simulink library "LM_LIB"  (R2019b)
settings: Solver=VariableStepAuto  StartTime=0.0  StopTime=10.0  RelTol=1e-3
undefined symbols (not defined in the file): P_LM_FusBLParFiltP, P_LM_FusParC0Index, P_LM_FusParC1Index, P_LM_FusParC2Index, P_LM_FusParC3Index, P_LM_OTLBufTPMinPntNum, P_LM_OTLBufTPSPosMinDis, P_LM_OTLRearMaxDis, P_LM_OTLTPNum
libraries: simulink x84, $bdroot x3
(part 5 of 5)

== system LM_LIB/LM_OTLBufLostTPValidJudgeNew/If Action Subsystem/If Action Subsystem/If Action Subsystem ==
  LM_OTLBufSPPosK1 : Inport
  LM_OTLBufEPPosK1 : Inport  Port=2
  LM_OTLBufPNumK1 : Inport  Port=3
  Action Port : ActionPort  ActionPortLabel=if(u1 ~= 0)
  Constant1 : Constant  OutDataTypeStr=uint8
  LM_OTLBufLastTPValid : Outport
  LM_OTLBufLastPNum : Outport  Port=2
  LM_OTLBufLastSPPos : Outport  Port=3
  LM_OTLBufLastEPPos : Outport  Port=4
  wires:
  LM_OTLBufSPPosK1/1 -> LM_OTLBufLastSPPos/1  "LM_OTLBufLastSPPos"
  LM_OTLBufEPPosK1/1 -> LM_OTLBufLastEPPos/1  "LM_OTLBufLastEPPos"
  LM_OTLBufPNumK1/1 -> LM_OTLBufLastPNum/1  "LM_OTLBufLastPNum"
  Constant1/1 -> LM_OTLBufLastTPValid/1  "LM_OTLBufLastTPValid"

== system LM_LIB/LM_OTLBufLostTPValidJudgeNew/If Action Subsystem/If Action Subsystem/If Action Subsystem1 ==
  LM_OTLBufDxVectK1Adju : Inport
  LM_OTLBufLastPNumK1 : Inport  Port=2
  LM_OTLBufLastSPPosK1 : Inport  Port=3
  LM_OTLBufLastEPPosK1 : Inport  Port=4
  Action Port : ActionPort  ActionPortLabel=else
  LM_OTL_Last1ObjValidTPDisClac : Subsystem
  LM_OTL_Last2ObjTPValidJudge : Subsystem
  Subsystem2 : Subsystem
  LM_OTLBufLastTPValid : Outport
  LM_OTLBufLastPNum : Outport  Port=2
  LM_OTLBufLastSPPos : Outport  Port=3
  LM_OTLBufLastEPPos : Outport  Port=4
  wires:
  LM_OTLBufDxVectK1Adju/1 -> LM_OTL_Last1ObjValidTPDisClac/1(LM_OTLBufDxVectK1Adju)
  LM_OTLBufLastSPPosK1/1 -> Subsystem2/2(LM_OTLBufLastSPPosK1), LM_OTL_Last1ObjValidTPDisClac/2(LM_OTLBufLastSPPosK1)
  LM_OTLBufLastEPPosK1/1 -> Subsystem2/3(LM_OTLBufLastEPPosK1), LM_OTL_Last1ObjValidTPDisClac/3(LM_OTLBufLastEPPosK1)
  LM_OTL_Last1ObjValidTPDisClac/1(LM_OTLLast2ObjValidTPDis) -> LM_OTL_Last2ObjTPValidJudge/1(LM_OTLLast2ObjValidTPDis)
  LM_OTL_Last2ObjTPValidJudge/1(LM_OTLLast2ObjTPValid) -> Subsystem2/1(LM_OTLLast2ObjTPValid)
  LM_OTLBufLastPNumK1/1 -> Subsystem2/4(LM_OTLBufLastPNumK1)
  Subsystem2/1(LM_OTLBufLastTPValid) -> LM_OTLBufLastTPValid/1
  Subsystem2/2(LM_OTLBufLastPNum) -> LM_OTLBufLastPNum/1
  Subsystem2/3(LM_OTLBufLastSPPos) -> LM_OTLBufLastSPPos/1
  Subsystem2/4(LM_OTLBufLastEPPos) -> LM_OTLBufLastEPPos/1

== system LM_LIB/LM_OTLBufLostTPValidJudgeNew/If Action Subsystem/If Action Subsystem/LM_OTL_Last1ObjTPValidJudge ==
  LM_OTLLast1ObjValidTPDis : Inport
  Constant : Constant  Value=10  OutDataTypeStr=single
  Relational Operator : RelationalOperator  OutDataTypeStr=boolean  RndMeth=Simplest
  LM_OTLLast1ObjTPValid : Outport
  wires:
  Relational Operator/1 -> LM_OTLLast1ObjTPValid/1  "LM_OTLLast1ObjTPValid"
  Constant/1 -> Relational Operator/2
  LM_OTLLast1ObjValidTPDis/1 -> Relational Operator/1

== system LM_LIB/LM_OTLBufLostTPValidJudgeNew/If Action Subsystem/If Action Subsystem/LM_OTL_Last1ObjValidTPDisClac ==
  LM_OTLBufL1DxVectK1Adju : Inport
  LM_OTLBufSPPosK1 : Inport  Port=2
  LM_OTLBufEPPosK1 : Inport  Port=3
  Constant : Constant  Value=0  OutDataTypeStr=single
  Index Vector : MultiPortSwitch  Inputs=1
  Index Vector1 : MultiPortSwitch  Inputs=1
  Relational Operator : RelationalOperator  Operator=>  OutDataTypeStr=boolean  RndMeth=Simplest
  Saturation : Saturate  UpperLimit=80  LowerLimit=1
  Saturation1 : Saturate  UpperLimit=80  LowerLimit=1
  Subtract : Sum  Inputs=+-
  Switch : Switch  Criteria=u2 ~= 0
  LM_OTLLast1ObjValidTPDis : Outport
  wires:
  Relational Operator/1 -> Switch/2
  Switch/1 -> Subtract/2
  Index Vector1/1 -> Subtract/1  "EndDis"
  Index Vector/1 -> Switch/1, Relational Operator/1  "StartDis"
  LM_OTLBufEPPosK1/1 -> Saturation/1
  LM_OTLBufL1DxVectK1Adju/1 -> Index Vector1/2, Index Vector/2
  LM_OTLBufSPPosK1/1 -> Saturation1/1
  Subtract/1 -> LM_OTLLast1ObjValidTPDis/1  "LM_OTLLast1ObjValidTPDis"
  Constant/1 -> Relational Operator/2, Switch/3
  Saturation/1 -> Index Vector1/1
  Saturation1/1 -> Index Vector/1

== system LM_LIB/LM_OTLBufLostTPValidJudgeNew/If Action Subsystem/If Action Subsystem1/LM_OTL_Last1ObjTPValidJudge ==
  LM_OTLLast1ObjValidTPDis : Inport
  Constant : Constant  Value=10  OutDataTypeStr=single
  Relational Operator : RelationalOperator  OutDataTypeStr=boolean  RndMeth=Simplest
  LM_OTLLast1ObjTPValid : Outport
  wires:
  LM_OTLLast1ObjValidTPDis/1 -> Relational Operator/1
  Constant/1 -> Relational Operator/2
  Relational Operator/1 -> LM_OTLLast1ObjTPValid/1  "LM_OTLLast1ObjTPValid"

== system LM_LIB/LM_OTLBufLostTPValidJudgeNew/If Action Subsystem/If Action Subsystem1/LM_OTL_Last1ObjValidTPDisClac ==
  LM_OTLBufL1DxVectK1Adju : Inport
  LM_OTLBufSPPosK1 : Inport  Port=2
  LM_OTLBufEPPosK1 : Inport  Port=3
  Constant : Constant  Value=0  OutDataTypeStr=single
  Index Vector : MultiPortSwitch  Inputs=1
  Index Vector1 : MultiPortSwitch  Inputs=1
  Relational Operator : RelationalOperator  Operator=>  OutDataTypeStr=boolean  RndMeth=Simplest
  Saturation : Saturate  UpperLimit=80  LowerLimit=1
  Saturation1 : Saturate  UpperLimit=80  LowerLimit=1
  Subtract : Sum  Inputs=+-
  Switch : Switch  Criteria=u2 ~= 0
  LM_OTLLast1ObjValidTPDis : Outport
  wires:
  LM_OTLBufSPPosK1/1 -> Saturation1/1
  LM_OTLBufL1DxVectK1Adju/1 -> Index Vector1/2, Index Vector/2
  LM_OTLBufEPPosK1/1 -> Saturation/1
  Index Vector/1 -> Switch/1, Relational Operator/1  "StartDis"
  Constant/1 -> Relational Operator/2, Switch/3
  Relational Operator/1 -> Switch/2
  Index Vector1/1 -> Subtract/1  "EndDis"
  Switch/1 -> Subtract/2
  Subtract/1 -> LM_OTLLast1ObjValidTPDis/1  "LM_OTLLast1ObjValidTPDis"
  Saturation/1 -> Index Vector1/1
  Saturation1/1 -> Index Vector/1

== system LM_LIB/LM_OTLBufLostTPValidJudgeNew/If Action Subsystem/If Action Subsystem1/LM_OTL_LastObjInfoCalc ==
  LM_OTLLast1ObjTPValid : Inport
  LM_OTLBufSPPosK1 : Inport  Port=2
  LM_OTLBufEPPosK1 : Inport  Port=3
  LM_OTLBufPNumK1 : Inport  Port=4
  Constant1 : Constant  OutDataTypeStr=uint8
  Constant2 : Constant  Value=0  OutDataTypeStr=uint8
  Constant3 : Constant  Value=0  OutDataTypeStr=uint8
  Switch{,1..3} (4 alike) : Switch  Criteria=u2 ~= 0
  LM_OTLBufLastTPValid : Outport
  LM_OTLBufLastPNum : Outport  Port=2
  LM_OTLBufLastSPPos : Outport  Port=3
  LM_OTLBufLastEPPos : Outport  Port=4
  wires:
  LM_OTLLast1ObjTPValid/1 -> Switch3/2, Switch2/2, Switch/2, Switch1/2
  Constant2/1 -> Switch1/3
  Constant1/1 -> Switch1/1
  Switch1/1 -> LM_OTLBufLastTPValid/1  "LM_OTLBufLastTPValid"
  Switch/1 -> LM_OTLBufLastPNum/1  "LM_OTLBufLastPNum"
  LM_OTLBufPNumK1/1 -> Switch/1
  Constant3/1 -> Switch3/3, Switch2/3, Switch/3
  Switch2/1 -> LM_OTLBufLastSPPos/1  "LM_OTLBufLastSPPos"
  LM_OTLBufSPPosK1/1 -> Switch2/1
  Switch3/1 -> LM_OTLBufLastEPPos/1  "LM_OTLBufLastEPPos"
  LM_OTLBufEPPosK1/1 -> Switch3/1

== system LM_LIB/LM_OTL_Buf1InfoUpdate/LM_OTL_BufLe1StoreInfoCalc/LM_OTL_ObjSICCurLeObj1InBufLe1/LM_OTL_BufL1DxInfo ==
  LM_OTLCurLeLaObj1Dx : Inport
  LM_OTLCurLeLaObj1RcdFlg : Inport  Port=2
  Constant : Constant  Value=0  OutDataTypeStr=single
  Switch4 : Switch  Criteria=u2 ~= 0
  LM_OTLBufL1Objdx : Outport
  wires:
  LM_OTLCurLeLaObj1Dx/1 -> Switch4/1
  LM_OTLCurLeLaObj1RcdFlg/1 -> Switch4/2
  Switch4/1 -> LM_OTLBufL1Objdx/1  "LM_OTLBufL1Objdx"
  Constant/1 -> Switch4/3

== system LM_LIB/LM_OTL_Buf1InfoUpdate/LM_OTL_BufLe1StoreInfoCalc/LM_OTL_ObjSICCurLeObj1InBufLe1/LM_OTL_BufL1DyInfo ==
  LM_OTLCurLeLaObj1Dy : Inport
  LM_OTLCurLeLaObj1RcdFlg : Inport  Port=2
  Constant : Constant  Value=0  OutDataTypeStr=single
  Switch4 : Switch  Criteria=u2 ~= 0
  LM_OTLBufL1ObjDy : Outport
  wires:
  Constant/1 -> Switch4/3
  Switch4/1 -> LM_OTLBufL1ObjDy/1  "LM_OTLBufL1ObjDy"
  LM_OTLCurLeLaObj1Dy/1 -> Switch4/1
  LM_OTLCurLeLaObj1RcdFlg/1 -> Switch4/2

== system LM_LIB/LM_OTL_Buf1InfoUpdate/LM_OTL_BufLe1StoreInfoCalc/LM_OTL_ObjSICCurLeObj1InBufLe1/LM_OTL_BufL1EPInfo ==
  note: P_LM_OTLTPNum
  LM_OTLCurLeLaObj1RcdFlg : Inport
  LM_OTLBufL1EPPosK1 : Inport  Port=2
  Add : Sum
  Constant : Constant  OutDataTypeStr=uint8
  Constant1 : Constant  Value=P_LM_OTLTPNum  OutDataTypeStr=uint8
  Constant2 : Constant  OutDataTypeStr=uint8
  Relational Operator : RelationalOperator  Operator=>  OutDataTypeStr=boolean  RndMeth=Simplest
  Switch1 : Switch  Criteria=u2 ~= 0
  Switch4 : Switch  Criteria=u2 ~= 0
  LM_OTLBufL1EPPos : Outport
  wires:
  Constant/1 -> Add/2
  LM_OTLCurLeLaObj1RcdFlg/1 -> Switch4/2
  LM_OTLBufL1EPPosK1/1 -> Switch4/3, Add/1
  Switch1/1 -> LM_OTLBufL1EPPos/1  "LM_OTLBufL1EPPos"
  Relational Operator/1 -> Switch1/2
  Switch4/1 -> Switch1/3, Relational Operator/1
  Constant1/1 -> Relational Operator/2
  Constant2/1 -> Switch1/1
  Add/1 -> Switch4/1

== system LM_LIB/LM_OTL_Buf1InfoUpdate/LM_OTL_BufLe1StoreInfoCalc/LM_OTL_ObjSICCurLeObj1InBufLe1/LM_OTL_BufL1IDInfo ==
  LM_OTLCurLeLaObj1ID : Inport
  Signal Conversion : SignalConversion  OverrideOpt=off
  LM_OTLBufL1ObjID : Outport
  wires:
  LM_OTLCurLeLaObj1ID/1 -> Signal Conversion/1
  Signal Conversion/1 -> LM_OTLBufL1ObjID/1  "LM_OTLBufL1ObjID"

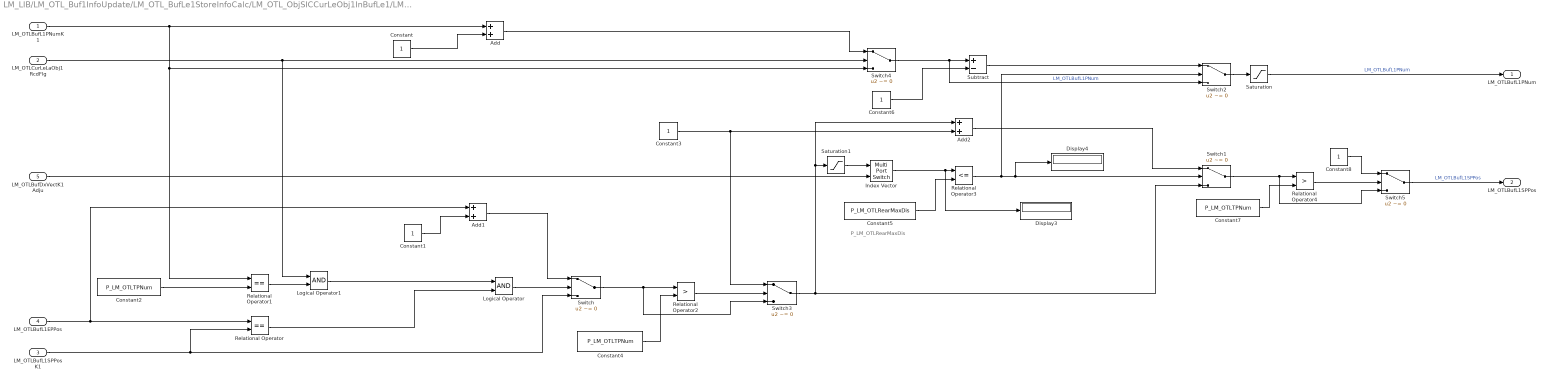
== system LM_LIB/LM_OTL_Buf1InfoUpdate/LM_OTL_BufLe1StoreInfoCalc/LM_OTL_ObjSICCurLeObj1InBufLe1/LM_OTL_BufL1PNumAndSPInfo ==
  note: P_LM_OTLRearMaxDis
  LM_OTLBufL1PNumK1 : Inport
  LM_OTLCurLeLaObj1RcdFlg : Inport  Port=2
  LM_OTLBufL1SPPosK1 : Inport  Port=3
  LM_OTLBufL1EPPos : Inport  Port=4
  LM_OTLBufDxVectK1Adju : Inport  Port=5
  Add : Sum
  Add1 : Sum
  Add2 : Sum
  Constant{,1,3,6,8} (5 alike) : Constant  OutDataTypeStr=uint8
  Constant2 : Constant  Value=P_LM_OTLTPNum  OutDataTypeStr=uint8
  Constant4 : Constant  Value=P_LM_OTLTPNum  OutDataTypeStr=uint8
  Constant5 : Constant  Value=P_LM_OTLRearMaxDis
  Constant7 : Constant  Value=P_LM_OTLTPNum  OutDataTypeStr=uint8
  Display3 : Display
  Display4 : Display
  Index Vector : MultiPortSwitch  Inputs=1
  Logical Operator : Logic  AllPortsSameDT=off  OutDataTypeStr=boolean
  Logical Operator1 : Logic  AllPortsSameDT=off  OutDataTypeStr=boolean
  Relational Operator : RelationalOperator  Operator===  OutDataTypeStr=boolean  RndMeth=Simplest
  Relational Operator1 : RelationalOperator  Operator===  OutDataTypeStr=boolean  RndMeth=Simplest
  Relational Operator2 : RelationalOperator  Operator=>  OutDataTypeStr=boolean  RndMeth=Simplest
  Relational Operator3 : RelationalOperator  Operator=<=  OutDataTypeStr=boolean  RndMeth=Simplest
  Relational Operator4 : RelationalOperator  Operator=>  OutDataTypeStr=boolean  RndMeth=Simplest
  Saturation : Saturate  UpperLimit=80  LowerLimit=0
  Saturation1 : Saturate  UpperLimit=80  LowerLimit=0
  Subtract : Sum  Inputs=+-
  Switch{,1..5} (6 alike) : Switch  Criteria=u2 ~= 0
  LM_OTLBufL1PNum : Outport
  LM_OTLBufL1SPPos : Outport  Port=2
  wires:
  Saturation/1 -> LM_OTLBufL1PNum/1  "LM_OTLBufL1PNum"
  LM_OTLCurLeLaObj1RcdFlg/1 -> Logical Operator1/1, Switch4/2
  Switch2/1 -> Saturation/1
  Constant/1 -> Add/2
  Add/1 -> Switch4/1
  Constant2/1 -> Relational Operator1/2
  Constant3/1 -> Switch3/1, Add2/2
  Constant4/1 -> Relational Operator2/2
  Add1/1 -> Switch/1
  Switch/1 -> Switch3/3, Relational Operator2/1
  Relational Operator2/1 -> Switch3/2
  LM_OTLBufL1SPPosK1/1 -> Switch/3, Relational Operator/2
  Relational Operator1/1 -> Logical Operator1/2
  Logical Operator/1 -> Switch/2
  LM_OTLBufL1EPPos/1 -> Relational Operator/1, Add1/1
  Relational Operator/1 -> Logical Operator/2
  LM_OTLBufL1PNumK1/1 -> Add/1, Relational Operator1/1, Switch4/3
  Switch3/1 -> Switch1/3, Add2/1, Saturation1/1
  Constant1/1 -> Add1/2
  LM_OTLBufDxVectK1Adju/1 -> Index Vector/2
  Index Vector/1 -> Display3/1, Relational Operator3/1
  Constant5/1 -> Relational Operator3/2
  Relational Operator3/1 -> Switch2/2, Display4/1, Switch1/2
  Switch5/1 -> LM_OTLBufL1SPPos/1  "LM_OTLBufL1SPPos"
  Add2/1 -> Switch1/1
  Subtract/1 -> Switch2/1
  Saturation1/1 -> Index Vector/1
  Logical Operator1/1 -> Logical Operator/1
  Switch4/1 -> Switch2/3, Subtract/1  "LM_OTLBufL1PNum"
  Constant6/1 -> Subtract/2
  Switch1/1 -> Switch5/3, Relational Operator4/1
  Relational Operator4/1 -> Switch5/2
  Constant7/1 -> Relational Operator4/2
  Constant8/1 -> Switch5/1

== system LM_LIB/LM_OTL_Buf1InfoUpdate/LM_OTL_BufLe1StoreInfoCalc/LM_OTL_ObjSICCurLeObj1InBufLe1/LM_OTL_BufL1UpdateFlg ==
  LM_OTLCurLeLaObj1RcdFlg : Inport
  Signal Conversion : SignalConversion  OverrideOpt=off
  LM_OTLBufL1UpdateFlg : Outport
  wires:
  LM_OTLCurLeLaObj1RcdFlg/1 -> Signal Conversion/1
  Signal Conversion/1 -> LM_OTLBufL1UpdateFlg/1  "LM_OTLBufL1UpdateFlg"

== system LM_LIB/LM_OTL_Buf1InfoUpdate/LM_OTL_BufLe1StoreInfoCalc/LM_OTL_ObjSICCurLeObj2InBufLe1/LM_OTL_BufL1DxInfo ==
  LM_OTLCurLeLaObj1Dx : Inport
  LM_OTLCurLeLaObj1RcdFlg : Inport  Port=2
  Constant : Constant  Value=0  OutDataTypeStr=single
  Switch4 : Switch  Criteria=u2 ~= 0
  LM_OTLBufL1Objdx : Outport
  wires:
  LM_OTLCurLeLaObj1Dx/1 -> Switch4/1
  LM_OTLCurLeLaObj1RcdFlg/1 -> Switch4/2
  Switch4/1 -> LM_OTLBufL1Objdx/1  "LM_OTLBufL1Objdx"
  Constant/1 -> Switch4/3

== system LM_LIB/LM_OTL_Buf1InfoUpdate/LM_OTL_BufLe1StoreInfoCalc/LM_OTL_ObjSICCurLeObj2InBufLe1/LM_OTL_BufL1DyInfo ==
  LM_OTLCurLeLaObj1Dy : Inport
  LM_OTLCurLeLaObj1RcdFlg : Inport  Port=2
  Constant : Constant  Value=0  OutDataTypeStr=single
  Switch4 : Switch  Criteria=u2 ~= 0
  LM_OTLBufL1ObjDy : Outport
  wires:
  Constant/1 -> Switch4/3
  Switch4/1 -> LM_OTLBufL1ObjDy/1  "LM_OTLBufL1ObjDy"
  LM_OTLCurLeLaObj1Dy/1 -> Switch4/1
  LM_OTLCurLeLaObj1RcdFlg/1 -> Switch4/2

== system LM_LIB/LM_OTL_Buf1InfoUpdate/LM_OTL_BufLe1StoreInfoCalc/LM_OTL_ObjSICCurLeObj2InBufLe1/LM_OTL_BufL1EPInfo ==
  note: P_LM_OTLTPNum
  LM_OTLCurLeLaObj1RcdFlg : Inport
  LM_OTLBufL1EPPosK1 : Inport  Port=2
  Add : Sum
  Constant : Constant  OutDataTypeStr=uint8
  Constant1 : Constant  Value=80  OutDataTypeStr=uint8
  Constant2 : Constant  OutDataTypeStr=uint8
  Relational Operator : RelationalOperator  Operator=>  OutDataTypeStr=boolean  RndMeth=Simplest
  Switch1 : Switch  Criteria=u2 ~= 0
  Switch4 : Switch  Criteria=u2 ~= 0
  LM_OTLBufL1EPPos : Outport
  wires:
  Constant/1 -> Add/2
  LM_OTLCurLeLaObj1RcdFlg/1 -> Switch4/2
  LM_OTLBufL1EPPosK1/1 -> Switch4/3, Add/1
  Switch1/1 -> LM_OTLBufL1EPPos/1  "LM_OTLBufL1EPPos"
  Relational Operator/1 -> Switch1/2
  Switch4/1 -> Switch1/3, Relational Operator/1
  Constant1/1 -> Relational Operator/2
  Constant2/1 -> Switch1/1
  Add/1 -> Switch4/1

== system LM_LIB/LM_OTL_Buf1InfoUpdate/LM_OTL_BufLe1StoreInfoCalc/LM_OTL_ObjSICCurLeObj2InBufLe1/LM_OTL_BufL1IDInfo ==
  LM_OTLCurLeLaObj1ID : Inport
  Signal Conversion : SignalConversion  OverrideOpt=off
  LM_OTLBufL1ObjID : Outport
  wires:
  LM_OTLCurLeLaObj1ID/1 -> Signal Conversion/1
  Signal Conversion/1 -> LM_OTLBufL1ObjID/1  "LM_OTLBufL1ObjID"

== system LM_LIB/LM_OTL_Buf1InfoUpdate/LM_OTL_BufLe1StoreInfoCalc/LM_OTL_ObjSICCurLeObj2InBufLe1/LM_OTL_BufL1PNumAndSPInfo ==
  note: P_LM_OTLRearMaxDis
  LM_OTLBufL1PNumK1 : Inport
  LM_OTLCurLeLaObj2RcdFlg : Inport  Port=2
  LM_OTLBufL1SPPosK1 : Inport  Port=3
  LM_OTLBufL1EPPos : Inport  Port=4
  LM_OTLBufDxVectK1Adju : Inport  Port=5
  Add : Sum
  Add1 : Sum
  Add2 : Sum
  Constant{,1,3,7} (4 alike) : Constant  OutDataTypeStr=uint8
  Constant2 : Constant  Value=P_LM_OTLTPNum  OutDataTypeStr=uint8
  Constant4 : Constant  Value=P_LM_OTLTPNum  OutDataTypeStr=uint8
  Constant5 : Constant  Value=P_LM_OTLRearMaxDis
  Constant6 : Constant  Value=P_LM_OTLTPNum  OutDataTypeStr=uint8
  Index Vector : MultiPortSwitch  Inputs=1
  Logical Operator : Logic  AllPortsSameDT=off  OutDataTypeStr=boolean
  Logical Operator1 : Logic  AllPortsSameDT=off  OutDataTypeStr=boolean
  Relational Operator : RelationalOperator  Operator===  OutDataTypeStr=boolean  RndMeth=Simplest
  Relational Operator1 : RelationalOperator  Operator===  OutDataTypeStr=boolean  RndMeth=Simplest
  Relational Operator2 : RelationalOperator  Operator=>  OutDataTypeStr=boolean  RndMeth=Simplest
  Relational Operator3 : RelationalOperator  Operator=<=  OutDataTypeStr=boolean  RndMeth=Simplest
  Relational Operator4 : RelationalOperator  Operator=>  OutDataTypeStr=boolean  RndMeth=Simplest
  Saturation : Saturate  UpperLimit=80  LowerLimit=0
  Saturation1 : Saturate  UpperLimit=80  LowerLimit=1
  Subtract : Sum  Inputs=+-
  Switch{,1..5} (6 alike) : Switch  Criteria=u2 ~= 0
  LM_OTLBufL1PNum : Outport
  LM_OTLBufL1SPPos : Outport  Port=2
  wires:
  Switch5/1 -> LM_OTLBufL1SPPos/1  "LM_OTLBufL1SPPos"
  LM_OTLBufL1PNumK1/1 -> Add/1, Switch4/3, Relational Operator1/1
  LM_OTLBufL1SPPosK1/1 -> Switch/3, Relational Operator/2
  Relational Operator2/1 -> Switch3/2
  Switch/1 -> Switch3/3, Relational Operator2/1
  Constant3/1 -> Add2/2, Switch3/1
  Relational Operator/1 -> Logical Operator/2
  Add1/1 -> Switch/1
  Relational Operator1/1 -> Logical Operator1/2
  Relational Operator3/1 -> Switch2/2, Switch1/2
  Add2/1 -> Switch1/1
  Index Vector/1 -> Relational Operator3/1
  LM_OTLBufL1EPPos/1 -> Relational Operator/1, Add1/1
  Constant1/1 -> Add1/2
  Constant/1 -> Subtract/2, Add/2
  LM_OTLCurLeLaObj2RcdFlg/1 -> Logical Operator1/1, Switch4/2
  Saturation/1 -> LM_OTLBufL1PNum/1  "LM_OTLBufL1PNum"
  Constant4/1 -> Relational Operator2/2
  Constant5/1 -> Relational Operator3/2
  Switch3/1 -> Switch1/3, Add2/1, Saturation1/1
  LM_OTLBufDxVectK1Adju/1 -> Index Vector/2
  Logical Operator/1 -> Switch/2
  Subtract/1 -> Switch2/1
  Saturation1/1 -> Index Vector/1
  Constant2/1 -> Relational Operator1/2
  Logical Operator1/1 -> Logical Operator/1
  Add/1 -> Switch4/1
  Switch2/1 -> Saturation/1  "LM_OTLBufL1PNum"
  Switch4/1 -> Subtract/1, Switch2/3  "LM_OTLBufL1PNum"
  Switch1/1 -> Switch5/3, Relational Operator4/1
  Relational Operator4/1 -> Switch5/2
  Constant6/1 -> Relational Operator4/2
  Constant7/1 -> Switch5/1

== system LM_LIB/LM_OTL_Buf1InfoUpdate/LM_OTL_BufLe1StoreInfoCalc/LM_OTL_ObjSICCurLeObj2InBufLe1/LM_OTL_BufL1UpdateFlg ==
  LM_OTLCurLeLaObj1RcdFlg : Inport
  Signal Conversion : SignalConversion  OverrideOpt=off
  LM_OTLBufL1UpdateFlg : Outport
  wires:
  LM_OTLCurLeLaObj1RcdFlg/1 -> Signal Conversion/1
  Signal Conversion/1 -> LM_OTLBufL1UpdateFlg/1  "LM_OTLBufL1UpdateFlg"

== system LM_LIB/LM_OTL_Buf1InfoUpdate/LM_OTL_BufLe1StoreInfoCalc/LM_OTL_ObjSICNoCurObjInBufLe1/LM_OTL_BufL1DxInfo ==
  LM_OTLCurLeLaObj1Index : Inport
  LM_OTLCurLeLaObj2Index : Inport  Port=2
  LM_OTLCurLeLaObj1RcdedFlg : Inport  Port=3
  LM_OTLCurLeLaObj1Dx : Inport  Port=4
  LM_OTLCurLeLaObj2Dx : Inport  Port=5
  Compare To Zero : simulink/Logic and Bit Operations/Compare To Zero  relop===  OutDataTypeStr=boolean
  Compare To Zero1 : simulink/Logic and Bit Operations/Compare To Zero  relop===  OutDataTypeStr=boolean
  Compare To Zero2 : simulink/Logic and Bit Operations/Compare To Zero  relop===  OutDataTypeStr=boolean
  Constant : Constant  Value=0  OutDataTypeStr=single
  Constant1 : Constant  Value=0  OutDataTypeStr=single
  DocBlock : simulink/Model-Wide Utilities/DocBlock  DocumentType=Text
      content=|
      | 1. 功能描述
      |    该模块主要功能
      | 2. 算法说明
      | 2.1 当左车道最近目标索引为0时，即左车道无目标，输出0
      | 2.2 当左车道最近目标索引不为0时
      |     2.2.1 如果左车道最近目标ID未在buffer中存储，则输出左车道最近目标的dx
      |     2.2.2 如果左车道最近目标ID已经在buffer中存储
      |           2.2.2.1 如果左车道第二近目标ID不为0，则输出左车道第二近目标dx
      |           2.2.2.2 如果左车道第二近目标ID为0，则输出0
  Switch1 : Switch  Criteria=u2 ~= 0
  Switch2 : Switch  Criteria=u2 ~= 0
  Switch4 : Switch  Criteria=u2 ~= 0
  LM_OTLBufL1Objdx : Outport
  wires:
  LM_OTLCurLeLaObj1RcdedFlg/1 -> Compare To Zero1/1
  Switch1/1 -> Switch4/3
  Switch4/1 -> LM_OTLBufL1Objdx/1  "LM_OTLBufL1Objdx"
  LM_OTLCurLeLaObj1Index/1 -> Compare To Zero/1
  LM_OTLCurLeLaObj2Index/1 -> Compare To Zero2/1
  Compare To Zero/1 -> Switch4/2
  Constant/1 -> Switch4/1
  Compare To Zero1/1 -> Switch1/2
  LM_OTLCurLeLaObj1Dx/1 -> Switch1/1
  Compare To Zero2/1 -> Switch2/2
  Constant1/1 -> Switch2/1
  Switch2/1 -> Switch1/3
  LM_OTLCurLeLaObj2Dx/1 -> Switch2/3

== system LM_LIB/LM_OTL_Buf1InfoUpdate/LM_OTL_BufLe1StoreInfoCalc/LM_OTL_ObjSICNoCurObjInBufLe1/LM_OTL_BufL1DyInfo ==
  LM_OTLCurLeLaObj1Index : Inport
  LM_OTLCurLeLaObj2Index : Inport  Port=2
  LM_OTLCurLeLaObj1RcdedFlg : Inport  Port=3
  LM_OTLCurLeLaObj1Dy : Inport  Port=4
  LM_OTLCurLeLaObj2Dy : Inport  Port=5
  Compare To Zero : simulink/Logic and Bit Operations/Compare To Zero  relop===  OutDataTypeStr=boolean
  Compare To Zero1 : simulink/Logic and Bit Operations/Compare To Zero  relop===  OutDataTypeStr=boolean
  Compare To Zero2 : simulink/Logic and Bit Operations/Compare To Zero  relop===  OutDataTypeStr=boolean
  Constant : Constant  Value=0  OutDataTypeStr=single
  Constant1 : Constant  Value=0  OutDataTypeStr=single
  Switch1 : Switch  Criteria=u2 ~= 0
  Switch2 : Switch  Criteria=u2 ~= 0
  Switch4 : Switch  Criteria=u2 ~= 0
  LM_OTLBufL1Objdy : Outport
  wires:
  Constant/1 -> Switch4/1
  LM_OTLCurLeLaObj1Dy/1 -> Switch1/1
  Compare To Zero1/1 -> Switch1/2
  LM_OTLCurLeLaObj1Index/1 -> Compare To Zero/1
  Switch1/1 -> Switch4/3
  Switch4/1 -> LM_OTLBufL1Objdy/1  "LM_OTLBufL1Objdy"
  Compare To Zero/1 -> Switch4/2
  Constant1/1 -> Switch2/1
  LM_OTLCurLeLaObj1RcdedFlg/1 -> Compare To Zero1/1
  LM_OTLCurLeLaObj2Index/1 -> Compare To Zero2/1
  LM_OTLCurLeLaObj2Dy/1 -> Switch2/3
  Compare To Zero2/1 -> Switch2/2
  Switch2/1 -> Switch1/3

== system LM_LIB/LM_OTL_Buf1InfoUpdate/LM_OTL_BufLe1StoreInfoCalc/LM_OTL_ObjSICNoCurObjInBufLe1/LM_OTL_BufL1EPInfo ==
  LM_OTLBufL1SPPos : Inport
  Signal Conversion : SignalConversion  OverrideOpt=off
  LM_OTLBufL1EPPos : Outport
  wires:
  Signal Conversion/1 -> LM_OTLBufL1EPPos/1  "LM_OTLBufL1EPPos"
  LM_OTLBufL1SPPos/1 -> Signal Conversion/1

== system LM_LIB/LM_OTL_Buf1InfoUpdate/LM_OTL_BufLe1StoreInfoCalc/LM_OTL_ObjSICNoCurObjInBufLe1/LM_OTL_BufL1IDInfo ==
  LM_OTLCurLeLaObj1Index : Inport
  LM_OTLCurLeLaObj2Index : Inport  Port=2
  LM_OTLCurLeLaObj1RcdedFlg : Inport  Port=3
  LM_OTLCurLeLaObj1ID : Inport  Port=4
  LM_OTLCurLeLaObj2ID : Inport  Port=5
  Compare To Zero : simulink/Logic and Bit Operations/Compare To Zero  relop===  OutDataTypeStr=boolean
  Compare To Zero1 : simulink/Logic and Bit Operations/Compare To Zero  relop===  OutDataTypeStr=boolean
  Compare To Zero2 : simulink/Logic and Bit Operations/Compare To Zero  relop===  OutDataTypeStr=boolean
  Compare To Zero3 : simulink/Logic and Bit Operations/Compare To Zero  relop=~=  OutDataTypeStr=boolean
  Constant : Constant  Value=0  OutDataTypeStr=single
  Constant1 : Constant  Value=0  OutDataTypeStr=single
  Switch1 : Switch  Criteria=u2 ~= 0
  Switch2 : Switch  Criteria=u2 ~= 0
  Switch4 : Switch  Criteria=u2 ~= 0
  LM_OTLBufL1UpdateFlg : Outport
  LM_OTLBufL1ObjID : Outport  Port=2
  wires:
  Constant/1 -> Switch4/1
  LM_OTLCurLeLaObj1ID/1 -> Switch1/1
  Compare To Zero1/1 -> Switch1/2
  LM_OTLCurLeLaObj1Index/1 -> Compare To Zero/1
  Switch1/1 -> Switch4/3
  Switch4/1 -> Compare To Zero3/1, LM_OTLBufL1ObjID/1  "LM_OTLBufL1ObjID"
  Compare To Zero/1 -> Switch4/2
  Constant1/1 -> Switch2/1
  LM_OTLCurLeLaObj1RcdedFlg/1 -> Compare To Zero1/1
  LM_OTLCurLeLaObj2Index/1 -> Compare To Zero2/1
  LM_OTLCurLeLaObj2ID/1 -> Switch2/3
  Compare To Zero2/1 -> Switch2/2
  Switch2/1 -> Switch1/3
  Compare To Zero3/1 -> LM_OTLBufL1UpdateFlg/1

== system LM_LIB/LM_OTL_Buf1InfoUpdate/LM_OTL_BufLe1StoreInfoCalc/LM_OTL_ObjSICNoCurObjInBufLe1/LM_OTL_BufL1PNumInfo ==
  LM_OTLCurLeLaObj1Index : Inport
  LM_OTLCurLeLaObj2Index : Inport  Port=2
  LM_OTLCurLeLaObj1RcdedFlg : Inport  Port=3
  Compare To Zero : simulink/Logic and Bit Operations/Compare To Zero  relop===  OutDataTypeStr=boolean
  Compare To Zero1 : simulink/Logic and Bit Operations/Compare To Zero  relop===  OutDataTypeStr=boolean
  Compare To Zero2 : simulink/Logic and Bit Operations/Compare To Zero  relop===  OutDataTypeStr=boolean
  Constant : Constant  Value=0  OutDataTypeStr=uint8
  Constant1 : Constant  Value=0  OutDataTypeStr=uint8
  Constant2 : Constant  OutDataTypeStr=uint8
  Constant3 : Constant  OutDataTypeStr=uint8
  Switch1 : Switch  Criteria=u2 ~= 0
  Switch2 : Switch  Criteria=u2 ~= 0
  Switch4 : Switch  Criteria=u2 ~= 0
  LM_OTLBufL1TPNum : Outport
  wires:
  Switch2/1 -> Switch1/3
  Switch4/1 -> LM_OTLBufL1TPNum/1  "LM_OTLBufL1TPNum"
  Compare To Zero2/1 -> Switch2/2
  Switch1/1 -> Switch4/3
  LM_OTLCurLeLaObj1RcdedFlg/1 -> Compare To Zero1/1
  LM_OTLCurLeLaObj2Index/1 -> Compare To Zero2/1
  LM_OTLCurLeLaObj1Index/1 -> Compare To Zero/1
  Constant1/1 -> Switch2/1
  Compare To Zero1/1 -> Switch1/2
  Constant/1 -> Switch4/1
  Compare To Zero/1 -> Switch4/2
  Constant2/1 -> Switch1/1
  Constant3/1 -> Switch2/3

== system LM_LIB/LM_OTL_Buf1InfoUpdate/LM_OTL_BufLe1StoreInfoCalc/LM_OTL_ObjSICNoCurObjInBufLe1/LM_OTL_BufL1SPInfo ==
  LM_OTLCurLeLaObj1Index : Inport
  LM_OTLCurLeLaObj2Index : Inport  Port=2
  LM_OTLCurLeLaObj1RcdedFlg : Inport  Port=3
  LM_OTLBufL1LastTPValid : Inport  Port=4
  LM_OTLBufL1LastEPPos : Inport  Port=5
  Add : Sum
  Compare To Zero{,1..3} (4 alike) : simulink/Logic and Bit Operations/Compare To Zero  relop===  OutDataTypeStr=boolean
  Constant : Constant  Value=0  OutDataTypeStr=uint8
  Constant1 : Constant  Value=0  OutDataTypeStr=uint8
  Constant2 : Constant  OutDataTypeStr=uint8
  Constant3 : Constant  OutDataTypeStr=uint8
  Constant4 : Constant  Value=P_LM_OTLTPNum  OutDataTypeStr=uint8
  Relational Operator2 : RelationalOperator  Operator=>  OutDataTypeStr=boolean  RndMeth=Simplest
  Switch{,1..4} (5 alike) : Switch  Criteria=u2 ~= 0
  LM_OTLBufL1SPPos : Outport
  wires:
  Constant/1 -> Switch4/1
  Compare To Zero/1 -> Switch4/2
  Constant1/1 -> Switch2/1
  Compare To Zero1/1 -> Switch1/2
  LM_OTLCurLeLaObj2Index/1 -> Compare To Zero2/1
  Switch1/1 -> Switch4/3
  LM_OTLCurLeLaObj1RcdedFlg/1 -> Compare To Zero1/1
  LM_OTLCurLeLaObj1Index/1 -> Compare To Zero/1
  Compare To Zero2/1 -> Switch2/2
  Switch3/1 -> LM_OTLBufL1SPPos/1  "LM_OTLBufL1SPPos"
  Switch/1 -> Switch1/1
  Switch2/1 -> Switch1/3
  Add/1 -> Switch2/3, Switch/3
  LM_OTLBufL1LastTPValid/1 -> Compare To Zero3/1
  Compare To Zero3/1 -> Switch/2
  Constant2/1 -> Add/2, Switch/1
  LM_OTLBufL1LastEPPos/1 -> Add/1
  Relational Operator2/1 -> Switch3/2
  Constant3/1 -> Switch3/1
  Switch4/1 -> Switch3/3, Relational Operator2/1
  Constant4/1 -> Relational Operator2/2

== system LM_LIB/LM_OTL_Buf2InfoUpdate/LM_OTL_BufLe1StoreInfoCalc/LM_OTL_ObjSICCurLeObj1InBufLe1/LM_OTL_BufL1DxInfo ==
  LM_OTLCurLeLaObj1Dx : Inport
  LM_OTLCurLeLaObj1RcdFlg : Inport  Port=2
  Constant : Constant  Value=0  OutDataTypeStr=single
  Switch4 : Switch  Criteria=u2 ~= 0
  LM_OTLBufL1Objdx : Outport
  wires:
  LM_OTLCurLeLaObj1Dx/1 -> Switch4/1
  LM_OTLCurLeLaObj1RcdFlg/1 -> Switch4/2
  Switch4/1 -> LM_OTLBufL1Objdx/1  "LM_OTLBufL1Objdx"
  Constant/1 -> Switch4/3

== system LM_LIB/LM_OTL_Buf2InfoUpdate/LM_OTL_BufLe1StoreInfoCalc/LM_OTL_ObjSICCurLeObj1InBufLe1/LM_OTL_BufL1DyInfo ==
  LM_OTLCurLeLaObj1Dy : Inport
  LM_OTLCurLeLaObj1RcdFlg : Inport  Port=2
  Constant : Constant  Value=0  OutDataTypeStr=single
  Switch4 : Switch  Criteria=u2 ~= 0
  LM_OTLBufL1ObjDy : Outport
  wires:
  Constant/1 -> Switch4/3
  Switch4/1 -> LM_OTLBufL1ObjDy/1  "LM_OTLBufL1ObjDy"
  LM_OTLCurLeLaObj1Dy/1 -> Switch4/1
  LM_OTLCurLeLaObj1RcdFlg/1 -> Switch4/2

== system LM_LIB/LM_OTL_Buf2InfoUpdate/LM_OTL_BufLe1StoreInfoCalc/LM_OTL_ObjSICCurLeObj1InBufLe1/LM_OTL_BufL1EPInfo ==
  note: P_LM_OTLTPNum
  LM_OTLCurLeLaObj1RcdFlg : Inport
  LM_OTLBufL1EPPosK1 : Inport  Port=2
  Add : Sum
  Constant : Constant  OutDataTypeStr=uint8
  Constant1 : Constant  Value=80  OutDataTypeStr=uint8
  Constant2 : Constant  OutDataTypeStr=uint8
  Relational Operator : RelationalOperator  Operator=>  OutDataTypeStr=boolean  RndMeth=Simplest
  Switch1 : Switch  Criteria=u2 ~= 0
  Switch4 : Switch  Criteria=u2 ~= 0
  LM_OTLBufL1EPPos : Outport
  wires:
  Constant/1 -> Add/2
  LM_OTLCurLeLaObj1RcdFlg/1 -> Switch4/2
  LM_OTLBufL1EPPosK1/1 -> Switch4/3, Add/1
  Switch4/1 -> LM_OTLBufL1EPPos/1  "LM_OTLBufL1EPPos"
  Switch1/1 -> Switch4/1
  Relational Operator/1 -> Switch1/2
  Add/1 -> Switch1/3, Relational Operator/1
  Constant1/1 -> Relational Operator/2
  Constant2/1 -> Switch1/1

== system LM_LIB/LM_OTL_Buf2InfoUpdate/LM_OTL_BufLe1StoreInfoCalc/LM_OTL_ObjSICCurLeObj1InBufLe1/LM_OTL_BufL1IDInfo ==
  LM_OTLCurLeLaObj1ID : Inport
  Signal Conversion : SignalConversion  OverrideOpt=off
  LM_OTLBufL1ObjID : Outport
  wires:
  LM_OTLCurLeLaObj1ID/1 -> Signal Conversion/1
  Signal Conversion/1 -> LM_OTLBufL1ObjID/1  "LM_OTLBufL1ObjID"

== system LM_LIB/LM_OTL_Buf2InfoUpdate/LM_OTL_BufLe1StoreInfoCalc/LM_OTL_ObjSICCurLeObj1InBufLe1/LM_OTL_BufL1UpdateFlg ==
  LM_OTLCurLeLaObj1RcdFlg : Inport
  Signal Conversion : SignalConversion  OverrideOpt=off
  LM_OTLBufL1UpdateFlg : Outport
  wires:
  LM_OTLCurLeLaObj1RcdFlg/1 -> Signal Conversion/1
  Signal Conversion/1 -> LM_OTLBufL1UpdateFlg/1  "LM_OTLBufL1UpdateFlg"

== system LM_LIB/LM_OTL_Buf2InfoUpdate/LM_OTL_BufLe1StoreInfoCalc/LM_OTL_ObjSICCurLeObj2InBufLe1/LM_OTL_BufL1DxInfo ==
  LM_OTLCurLeLaObj1Dx : Inport
  LM_OTLCurLeLaObj1RcdFlg : Inport  Port=2
  Constant : Constant  Value=0  OutDataTypeStr=single
  Switch4 : Switch  Criteria=u2 ~= 0
  LM_OTLBufL1Objdx : Outport
  wires:
  LM_OTLCurLeLaObj1Dx/1 -> Switch4/1
  LM_OTLCurLeLaObj1RcdFlg/1 -> Switch4/2
  Switch4/1 -> LM_OTLBufL1Objdx/1  "LM_OTLBufL1Objdx"
  Constant/1 -> Switch4/3

== system LM_LIB/LM_OTL_Buf2InfoUpdate/LM_OTL_BufLe1StoreInfoCalc/LM_OTL_ObjSICCurLeObj2InBufLe1/LM_OTL_BufL1DyInfo ==
  LM_OTLCurLeLaObj1Dy : Inport
  LM_OTLCurLeLaObj1RcdFlg : Inport  Port=2
  Constant : Constant  Value=0  OutDataTypeStr=single
  Switch4 : Switch  Criteria=u2 ~= 0
  LM_OTLBufL1ObjDy : Outport
  wires:
  Constant/1 -> Switch4/3
  Switch4/1 -> LM_OTLBufL1ObjDy/1  "LM_OTLBufL1ObjDy"
  LM_OTLCurLeLaObj1Dy/1 -> Switch4/1
  LM_OTLCurLeLaObj1RcdFlg/1 -> Switch4/2

== system LM_LIB/LM_OTL_Buf2InfoUpdate/LM_OTL_BufLe1StoreInfoCalc/LM_OTL_ObjSICCurLeObj2InBufLe1/LM_OTL_BufL1EPInfo ==
  note: P_LM_OTLTPNum
  LM_OTLCurLeLaObj1RcdFlg : Inport
  LM_OTLBufL1EPPosK1 : Inport  Port=2
  Add : Sum
  Constant : Constant  OutDataTypeStr=uint8
  Constant1 : Constant  Value=80  OutDataTypeStr=uint8
  Constant2 : Constant  OutDataTypeStr=uint8
  Relational Operator : RelationalOperator  Operator=>  OutDataTypeStr=boolean  RndMeth=Simplest
  Switch1 : Switch  Criteria=u2 ~= 0
  Switch4 : Switch  Criteria=u2 ~= 0
  LM_OTLBufL1EPPos : Outport
  wires:
  Constant/1 -> Add/2
  LM_OTLCurLeLaObj1RcdFlg/1 -> Switch4/2
  LM_OTLBufL1EPPosK1/1 -> Switch4/3, Add/1
  Switch4/1 -> LM_OTLBufL1EPPos/1  "LM_OTLBufL1EPPos"
  Switch1/1 -> Switch4/1
  Relational Operator/1 -> Switch1/2
  Add/1 -> Switch1/3, Relational Operator/1
  Constant1/1 -> Relational Operator/2
  Constant2/1 -> Switch1/1

== system LM_LIB/LM_OTL_Buf2InfoUpdate/LM_OTL_BufLe1StoreInfoCalc/LM_OTL_ObjSICCurLeObj2InBufLe1/LM_OTL_BufL1IDInfo ==
  LM_OTLCurLeLaObj1ID : Inport
  Signal Conversion : SignalConversion  OverrideOpt=off
  LM_OTLBufL1ObjID : Outport
  wires:
  LM_OTLCurLeLaObj1ID/1 -> Signal Conversion/1
  Signal Conversion/1 -> LM_OTLBufL1ObjID/1  "LM_OTLBufL1ObjID"

== system LM_LIB/LM_OTL_Buf2InfoUpdate/LM_OTL_BufLe1StoreInfoCalc/LM_OTL_ObjSICCurLeObj2InBufLe1/LM_OTL_BufL1UpdateFlg ==
  LM_OTLCurLeLaObj1RcdFlg : Inport
  Signal Conversion : SignalConversion  OverrideOpt=off
  LM_OTLBufL1UpdateFlg : Outport
  wires:
  LM_OTLCurLeLaObj1RcdFlg/1 -> Signal Conversion/1
  Signal Conversion/1 -> LM_OTLBufL1UpdateFlg/1  "LM_OTLBufL1UpdateFlg"

== system LM_LIB/LM_OTL_Buf2InfoUpdate/LM_OTL_BufLe1StoreInfoCalc/LM_OTL_ObjSICNoCurObjInBufLe1/LM_OTL_BufL1IDInfo ==
  LM_OTLBuf1ID : Inport
  LM_OTLCurLeLaObj1Index : Inport  Port=2
  LM_OTLCurLeLaObj2Index : Inport  Port=3
  LM_OTLCurLeLaObj1RcdedFlg : Inport  Port=4
  LM_OTLCurLeLaObj1ID : Inport  Port=5
  LM_OTLCurLeLaObj2ID : Inport  Port=6
  Compare To Zero : simulink/Logic and Bit Operations/Compare To Zero  relop===  OutDataTypeStr=boolean
  Compare To Zero1 : simulink/Logic and Bit Operations/Compare To Zero  relop===  OutDataTypeStr=boolean
  Compare To Zero2 : simulink/Logic and Bit Operations/Compare To Zero  relop===  OutDataTypeStr=boolean
  Compare To Zero3 : simulink/Logic and Bit Operations/Compare To Zero  relop=~=  OutDataTypeStr=boolean
  Constant : Constant  Value=0  OutDataTypeStr=single
  Constant1 : Constant  Value=0  OutDataTypeStr=single
  Relational Operator1 : RelationalOperator  Operator===  OutDataTypeStr=boolean  RndMeth=Simplest
  Switch{1..2,4..5} (4 alike) : Switch  Criteria=u2 ~= 0
  LM_OTLBufL2UpdateFlg : Outport
  LM_OTLBufL2ObjID : Outport  Port=2
  wires:
  Constant/1 -> Switch4/1
  LM_OTLCurLeLaObj1ID/1 -> Switch1/1
  Compare To Zero1/1 -> Switch1/2
  LM_OTLCurLeLaObj1Index/1 -> Compare To Zero/1
  Switch4/1 -> LM_OTLBufL2ObjID/1, Compare To Zero3/1  "LM_OTLBufL1ObjID"
  Compare To Zero/1 -> Switch4/2
  Constant1/1 -> Switch2/1
  LM_OTLCurLeLaObj1RcdedFlg/1 -> Compare To Zero1/1
  LM_OTLCurLeLaObj2Index/1 -> Compare To Zero2/1
  LM_OTLCurLeLaObj2ID/1 -> Switch2/3
  Compare To Zero2/1 -> Switch2/2
  Compare To Zero3/1 -> LM_OTLBufL2UpdateFlg/1
  Switch2/1 -> Switch5/1, Switch1/3
  LM_OTLBuf1ID/1 -> Relational Operator1/1
  Switch1/1 -> Switch5/3, Relational Operator1/2
  Relational Operator1/1 -> Switch5/2
  Switch5/1 -> Switch4/3  "LM_OTLBufL1ObjID"

== system LM_LIB/LM_OTL_Buf2InfoUpdate/LM_OTL_BufLe1StoreInfoCalc/LM_OTL_ObjSICNoCurObjInBufLe1/LM_OTL_BufL1PNumInfo ==
  LM_OTLBufL2ObjID : Inport
  Compare To Zero : simulink/Logic and Bit Operations/Compare To Zero  relop===  OutDataTypeStr=boolean
  Constant : Constant  Value=0  OutDataTypeStr=uint8
  Constant2 : Constant  OutDataTypeStr=uint8
  Switch4 : Switch  Criteria=u2 ~= 0
  LM_OTLBufL1TPNum : Outport
  wires:
  Switch4/1 -> LM_OTLBufL1TPNum/1  "LM_OTLBufL1TPNum"
  Constant2/1 -> Switch4/3
  LM_OTLBufL2ObjID/1 -> Compare To Zero/1
  Constant/1 -> Switch4/1
  Compare To Zero/1 -> Switch4/2

== system LM_LIB/LM_OTL_Buf2InfoUpdate/LM_OTL_BufLe1StoreInfoCalc/LM_OTL_ObjSICNoCurObjInBufLe1/LM_OTL_BufL1SPInfo ==
  LM_OTLBufL2ObjID : Inport
  LM_OTLBufL2LastTPValid : Inport  Port=2
  LM_OTLBufL2LastEPPos : Inport  Port=3
  Add : Sum
  Compare To Zero : simulink/Logic and Bit Operations/Compare To Zero  relop===  OutDataTypeStr=boolean
  Compare To Zero3 : simulink/Logic and Bit Operations/Compare To Zero  relop===  OutDataTypeStr=boolean
  Constant : Constant  Value=0  OutDataTypeStr=uint8
  Constant1 : Constant  OutDataTypeStr=uint8
  Constant2 : Constant  OutDataTypeStr=uint8
  Constant3 : Constant  Value=P_LM_OTLTPNum  OutDataTypeStr=uint8
  Relational Operator2 : RelationalOperator  Operator=>  OutDataTypeStr=boolean  RndMeth=Simplest
  Switch : Switch  Criteria=u2 ~= 0
  Switch1 : Switch  Criteria=u2 ~= 0
  Switch4 : Switch  Criteria=u2 ~= 0
  LM_OTLBufL2SPPos : Outport
  wires:
  Constant/1 -> Switch4/1
  Compare To Zero/1 -> Switch4/2
  Switch/1 -> Switch4/3
  LM_OTLBufL2ObjID/1 -> Compare To Zero/1
  Switch1/1 -> LM_OTLBufL2SPPos/1  "LM_OTLBufL2SPPos"
  Add/1 -> Switch/3
  LM_OTLBufL2LastTPValid/1 -> Compare To Zero3/1
  Compare To Zero3/1 -> Switch/2
  Constant2/1 -> Add/2, Switch/1
  LM_OTLBufL2LastEPPos/1 -> Add/1
  Constant1/1 -> Switch1/1
  Constant3/1 -> Relational Operator2/2
  Switch4/1 -> Switch1/3, Relational Operator2/1
  Relational Operator2/1 -> Switch1/2

== system LM_LIB/LM_OTL_Buf2InfoUpdate/LM_OTL_BufLe1StoreInfoCalc/LM_OTL_ObjSICNoCurObjInBufLe1/LM_OTL_BufL2EPInfo ==
  LM_OTLBufL2SPPos : Inport
  Signal Conversion : SignalConversion  OverrideOpt=off
  LM_OTLBufL2EPPos : Outport
  wires:
  Signal Conversion/1 -> LM_OTLBufL2EPPos/1  "LM_OTLBufL2EPPos"
  LM_OTLBufL2SPPos/1 -> Signal Conversion/1

== system LM_LIB/LM_OTL_Buf2InfoUpdate/LM_OTL_BufLe1StoreInfoCalc/LM_OTL_ObjSICNoCurObjInBufLe1/LM_OTL_BufL2PosInfo ==
  LM_OTLBufL2ObjID : Inport
  LM_OTLCurLeLaObj1ID : Inport  Port=2
  LM_OTLCurLeLaObj2ID : Inport  Port=3
  LM_OTLCurLeLaObj1Dx : Inport  Port=4
  LM_OTLCurLeLaObj2Dx : Inport  Port=5
  LM_OTLCurLeLaObj1Dy : Inport  Port=6
  LM_OTLCurLeLaObj2Dy : Inport  Port=7
  Compare To Zero : simulink/Logic and Bit Operations/Compare To Zero  relop===  OutDataTypeStr=boolean
  Constant : Constant  Value=0  OutDataTypeStr=single
  Constant1 : Constant  Value=0  OutDataTypeStr=single
  Constant2 : Constant  Value=0  OutDataTypeStr=single
  DocBlock : simulink/Model-Wide Utilities/DocBlock  DocumentType=Text
      content=|
      | 1. 功能描述
      |    该模块主要功能
      | 2. 算法说明
      | 2.1 当左车道最近目标索引为0时，即左车道无目标，输出0
      | 2.2 当左车道最近目标索引不为0时
      |     2.2.1 如果左车道最近目标ID未在buffer中存储，则输出左车道最近目标的dx
      |     2.2.2 如果左车道最近目标ID已经在buffer中存储
      |           2.2.2.1 如果左车道第二近目标ID不为0，则输出左车道第二近目标dx
      |           2.2.2.2 如果左车道第二近目标ID为0，则输出0
  Relational Operator : RelationalOperator  Operator===  OutDataTypeStr=boolean  RndMeth=Simplest
  Relational Operator1 : RelationalOperator  Operator===  OutDataTypeStr=boolean  RndMeth=Simplest
  Switch{1..6} (6 alike) : Switch  Criteria=u2 ~= 0
  LM_OTLBufL2Objdx : Outport
  LM_OTLBufL2Objdy : Outport  Port=2
  wires:
  Switch1/1 -> Switch4/3
  Switch4/1 -> LM_OTLBufL2Objdx/1  "LM_OTLBufL2Objdx"
  LM_OTLBufL2ObjID/1 -> Relational Operator/1, Relational Operator1/1, Compare To Zero/1
  Compare To Zero/1 -> Switch5/2, Switch4/2
  Constant/1 -> Switch5/1, Switch4/1
  LM_OTLCurLeLaObj1Dx/1 -> Switch1/1
  Relational Operator1/1 -> Switch6/2, Switch2/2
  LM_OTLCurLeLaObj2Dx/1 -> Switch2/1
  Switch2/1 -> Switch1/3
  LM_OTLCurLeLaObj1ID/1 -> Relational Operator/2
  Relational Operator/1 -> Switch3/2, Switch1/2
  LM_OTLCurLeLaObj2ID/1 -> Relational Operator1/2
  Constant1/1 -> Switch2/3
  LM_OTLCurLeLaObj1Dy/1 -> Switch3/1
  Switch3/1 -> Switch5/3
  LM_OTLCurLeLaObj2Dy/1 -> Switch6/1
  Switch6/1 -> Switch3/3
  Constant2/1 -> Switch6/3
  Switch5/1 -> LM_OTLBufL2Objdy/1  "LM_OTLBufL2Objdy"

== system LM_LIB/LM_OTLBufLostTPValidJudgeNew/If Action Subsystem/If Action Subsystem/If Action Subsystem1/LM_OTL_Last1ObjValidTPDisClac ==
  LM_OTLBufDxVectK1Adju : Inport
  LM_OTLBufLastSPPosK1 : Inport  Port=2
  LM_OTLBufLastEPPosK1 : Inport  Port=3
  Constant : Constant  Value=0  OutDataTypeStr=single
  Index Vector : MultiPortSwitch  Inputs=1
  Index Vector1 : MultiPortSwitch  Inputs=1
  Relational Operator : RelationalOperator  Operator=>  OutDataTypeStr=boolean  RndMeth=Simplest
  Saturation : Saturate  UpperLimit=80  LowerLimit=1
  Saturation1 : Saturate  UpperLimit=80  LowerLimit=1
  Subtract : Sum  Inputs=+-
  Switch : Switch  Criteria=u2 ~= 0
  LM_OTLLast2ObjValidTPDis : Outport
  wires:
  LM_OTLBufDxVectK1Adju/1 -> Index Vector1/2, Index Vector/2
  Subtract/1 -> LM_OTLLast2ObjValidTPDis/1  "LM_OTLLast2ObjValidTPDis"
  LM_OTLBufLastSPPosK1/1 -> Saturation1/1
  Constant/1 -> Relational Operator/2, Switch/3
  Index Vector/1 -> Switch/1, Relational Operator/1  "StartDis"
  Relational Operator/1 -> Switch/2
  Switch/1 -> Subtract/2
  LM_OTLBufLastEPPosK1/1 -> Saturation/1
  Index Vector1/1 -> Subtract/1  "EndDis"
  Saturation/1 -> Index Vector1/1
  Saturation1/1 -> Index Vector/1

== system LM_LIB/LM_OTLBufLostTPValidJudgeNew/If Action Subsystem/If Action Subsystem/If Action Subsystem1/LM_OTL_Last2ObjTPValidJudge ==
  LM_OTLLast2ObjValidTPDis : Inport
  Constant : Constant  Value=10  OutDataTypeStr=single
  Relational Operator : RelationalOperator  OutDataTypeStr=boolean  RndMeth=Simplest
  LM_OTLLast2ObjTPValid : Outport
  wires:
  LM_OTLLast2ObjValidTPDis/1 -> Relational Operator/1
  Relational Operator/1 -> LM_OTLLast2ObjTPValid/1  "LM_OTLLast2ObjTPValid"
  Constant/1 -> Relational Operator/2

== system LM_LIB/LM_OTLBufLostTPValidJudgeNew/If Action Subsystem/If Action Subsystem/If Action Subsystem1/Subsystem2 ==
  LM_OTLLast2ObjTPValid : Inport
  LM_OTLBufLastSPPosK1 : Inport  Port=2
  LM_OTLBufLastEPPosK1 : Inport  Port=3
  LM_OTLBufLastPNumK1 : Inport  Port=4
  Constant1 : Constant  OutDataTypeStr=uint8
  Constant2 : Constant  Value=0  OutDataTypeStr=uint8
  Constant3 : Constant  Value=0  OutDataTypeStr=uint8
  Switch{,1..3} (4 alike) : Switch  Criteria=u2 ~= 0
  LM_OTLBufLastTPValid : Outport
  LM_OTLBufLastPNum : Outport  Port=2
  LM_OTLBufLastSPPos : Outport  Port=3
  LM_OTLBufLastEPPos : Outport  Port=4
  wires:
  Switch2/1 -> LM_OTLBufLastSPPos/1  "LM_OTLBufLastSPPos"
  Constant3/1 -> Switch3/3, Switch2/3, Switch/3
  Constant2/1 -> Switch1/3
  Constant1/1 -> Switch1/1
  LM_OTLBufLastSPPosK1/1 -> Switch2/1
  Switch3/1 -> LM_OTLBufLastEPPos/1  "LM_OTLBufLastEPPos"
  LM_OTLBufLastEPPosK1/1 -> Switch3/1
  Switch/1 -> LM_OTLBufLastPNum/1  "LM_OTLBufLastPNum"
  Switch1/1 -> LM_OTLBufLastTPValid/1  "LM_OTLBufLastTPValid"
  LM_OTLLast2ObjTPValid/1 -> Switch3/2, Switch2/2, Switch/2, Switch1/2
  LM_OTLBufLastPNumK1/1 -> Switch/1

== matlab function LM_LIB/LM_OTLBuf2InfoNew/LM_OTL_BufLe1StoreInfoCalc/LM_OTL_ObjSICCurLeObj1InBufLe1/LM_OTL_BufL1DyInfo/MATLAB Function ==
  data: dx input; dyFilt output; dy input; varDy input; vy input; varVy input; psiDt input; tDt input; dyHist input; varDyHist input; varDyFilt output
function  [dyFilt,varDyFilt] = KF_Func(dx,dy,varDy,...
    vy,varVy,psiDt,tDt,dyHist,varDyHist)


ayManeuver = single(5);
vyAbs  = single(vy + (psiDt*dx));


% Calculate process noise: (0.5*a_maneuver*t^2)^2 */
q = (tDt*tDt) * (tDt*tDt);
q =q*(0.5 * ayManeuver)*(0.5 * ayManeuver);
% the following code caused problems on bit-identity: */
% q = (0.5 * CF_TRYFUS_ayManeuver) * (tDt*tDt); */
% q *=q; */

% retrodict current object data */
dyRetro    = dy - (vyAbs  * tDt);
varDyRetro = varDy  + ( (varVy * (tDt * tDt)) + q);

% filter retrodicted data with historical data */
K = varDyRetro / max(1e-6, (varDyRetro + varDyHist));

dyFilt    = single(((1.0 - K) * dyRetro)  +  (K * dyHist));
varDyFilt =  single((1.0 - K) * varDyRetro);

== matlab function LM_LIB/LM_OTLBuf2InfoNew/LM_OTL_BufLe1StoreInfoCalc/LM_OTL_ObjSICCurLeObj2InBufLe1/LM_OTL_BufL1DyInfo/MATLAB Function ==
  data: dx input; dyFilt output; dy input; varDy input; vy input; varVy input; psiDt input; tDt input; dyHist input; varDyHist input; varDyFilt output
function  [dyFilt,varDyFilt] = KF_Func(dx,dy,varDy,...
    vy,varVy,psiDt,tDt,dyHist,varDyHist)


ayManeuver = 5;
vyAbs  = vy + (psiDt*dx);


% Calculate process noise: (0.5*a_maneuver*t^2)^2 */
q = (tDt*tDt) * (tDt*tDt);
q =q*(0.5 * ayManeuver)*(0.5 * ayManeuver);
% the following code caused problems on bit-identity: */
% q = (0.5 * CF_TRYFUS_ayManeuver) * (tDt*tDt); */
% q *=q; */

% retrodict current object data */
dyRetro    = dy - (vyAbs  * tDt);
varDyRetro = varDy  + ( (varVy * (tDt * tDt)) + q);

% filter retrodicted data with historical data */
K = varDyRetro / max(1e-6, (varDyRetro + varDyHist));

dyFilt    = ((1.0 - K) * dyRetro)  +  (K * dyHist);
varDyFilt =  (1.0 - K) * varDyRetro;

== stateflow chart LM_LIB/LM_EVOFusPath/LM_FusBLPathQualityCalc ==
  state PathDisappear
    en:
    LM_FusBLPathQuality = single(0);
    du:
    LM_FusBLPathQuality = single(0);
    ex:
    LM_FusBLPathQuality = single(0);
  state PathMid2Appear
    en:
    t_times = uint8(0);
    LM_FusBLPathQuality = single(0);
    du:
    t_times = t_times + uint8(1);
    LM_FusBLPathQuality = single(0);
  state PathMid2Disappear
    en:
    t_times = uint8(0);
    LM_FusBLPathQuality = LM_FusPathEMLK * LM_EMLPathQuality + LM_FusPathVSLK * LM_VSLPathQuality + LM_FusPathOTLK * LM_OTLPathQuality;
    du:
    t_times = t_times + uint8(1);
    LM_FusBLPathQuality = LM_FusPathEMLK * LM_EMLPathQuality + LM_FusPathVSLK * LM_VSLPathQuality + LM_FusPathOTLK * LM_OTLPathQuality;
  state PathAppear
    en:
    LM_FusBLPathQuality = LM_FusPathEMLK * LM_EMLPathQuality + LM_FusPathVSLK * LM_VSLPathQuality + LM_FusPathOTLK * LM_OTLPathQuality;
    du:
    LM_FusBLPathQuality = LM_FusPathEMLK * LM_EMLPathQuality + LM_FusPathVSLK * LM_VSLPathQuality + LM_FusPathOTLK * LM_OTLPathQuality;
  (default) -> PathDisappear
  PathMid2Disappear -> PathDisappear [order 2] : [(LM_EMLPathQuality == 0 && LM_VSLPathQuality == 0 && LM_OTLPathQuality == 0) && t_times > 10]
  PathDisappear -> PathMid2Appear : [LM_EMLPathQuality ~= 0 || LM_VSLPathQuality ~= 0 || LM_OTLPathQuality ~= 0]
  PathMid2Appear -> PathDisappear [order 1] : [LM_EMLPathQuality == 0 && LM_VSLPathQuality == 0 && LM_OTLPathQuality == 0]
  PathMid2Appear -> PathAppear [order 2] : [(LM_EMLPathQuality ~= 0 || LM_VSLPathQuality ~= 0 || LM_OTLPathQuality ~= 0) && t_times > uint8(5)]
  PathMid2Disappear -> PathAppear [order 1] : [LM_EMLPathQuality ~= 0 || LM_VSLPathQuality ~= 0 || LM_OTLPathQuality ~= 0]
  PathAppear -> PathMid2Disappear : [LM_EMLPathQuality == 0 && LM_VSLPathQuality == 0 && LM_OTLPathQuality == 0]
  data: LM_EMLPathQuality input; LM_VSLPathQuality input; LM_OTLPathQuality input; LM_FusPathEMLK input; LM_FusPathVSLK input; LM_FusPathOTLK input; LM_FusBLPathQuality output single size=1; t_times local uint8 size=1

== stateflow chart LM_LIB/Chart2 ==
  state Lost
    en:LM_LINE_Filt = RFM_LINE;
    du:LM_LINE_Filt = RFM_LINE;
    ex:LM_LINE_Filt = LM_LINE_K1;
  state filt
    en:LM_LINE_Filt = LM_LINE_K1;
    existimes = uint8(0);
    du:
    existimes = existimes +uint8(1);
    LM_LINE_Filt = LM_LINE_K1;
    ex:LM_LINE_Filt = LM_LINE_K1;
  state Exist
    en:
    if abs(RFM_LINE.dC2V) <= 0.25 && abs(RFM_LINE.dC3V) <= 1 && abs(RFM_LINE.dC1V) <= 1
    LM_LINE_Filt = RFM_LINE；
    else
    LM_LINE_Filt = LM_LINE_K1;
    end
    du:
    if abs(RFM_LINE.dC2V) <= 0.25 && abs(RFM_LINE.dC3V) <= 1 && abs(RFM_LINE.dC1V) <= 1
    LM_LINE_Filt = RFM_LINE；
    if abs(RFM_LINE.dC2V-LM_LINE_K1.dC2V) <= 1 &&  abs(RFM_LINE.dC3V-LM_LINE_K1.dC3V) <= 1
    LM_LINE_Filt.dC0V=LM_LINE_K1.dC0V+0.75*(RFM_LINE.dC0V-LM_LINE_K1.dC0V);
    LM_LINE_Filt.dC1V=LM_LINE_K1.dC1V+0.75*(RFM_LINE.dC1V-LM_LINE_K1.dC1V);
    LM_LINE_Filt.dC2V=LM_LINE_K1.dC2V+0.15*(RFM_LINE.dC2V-LM_LINE_K1.dC2V);
    LM_LINE_Filt.dC3V=LM_LINE_K1.dC3V+0.15*(RFM_LINE.dC3V-LM_LINE_K1.dC3V);
    LM_LINE_Filt.dDisFront=LM_LINE_K1.dDisFront+0.15*(RFM_LINE.dDisFront-LM_LINE_K1.dDisFront);
    end
    else
    LM_LINE_Filt = LM_LINE_K1;
    end
  (default) -> Lost
  Lost -> filt : [RFM_LINE.bIsLineExist==2]
  Exist -> Lost : [RFM_LINE.bIsLineExist==1]
  filt -> Exist : [RFM_LINE.dQuality >= 0.1 && RFM_LINE.bIsLineExist==2 && existimes >25]
  data: RFM_LINE input Bus: RFM_LINE_BUS; LM_LINE_Filt output Bus: RFM_LINE_BUS size=1 =0; LM_LINE_K1 input Bus: RFM_LINE_BUS; existimes local uint8

== matlab function LM_LIB/LM_OTLBuf1InfoNew/LM_OTL_BufLe1StoreInfoCalc/LM_OTL_ObjSICCurLeObj1InBufLe1/LM_OTL_BufL1DyInfo/MATLAB Function ==
  data: dx input; dyFilt output; dy input; varDy input; vy input; varVy input; psiDt input; tDt input; dyHist input; varDyHist input; varDyFilt output
function  [dyFilt,varDyFilt] = KF_Func(dx,dy,varDy,...
    vy,varVy,psiDt,tDt,dyHist,varDyHist)


ayManeuver = 5;
vyAbs  = vy + (psiDt*dx);


% Calculate process noise: (0.5*a_maneuver*t^2)^2 */
q = (tDt*tDt) * (tDt*tDt);
q =q*(0.5 * ayManeuver)*(0.5 * ayManeuver);
% the following code caused problems on bit-identity: */
% q = (0.5 * CF_TRYFUS_ayManeuver) * (tDt*tDt); */
% q *=q; */

% retrodict current object data */
dyRetro    = dy - (vyAbs  * tDt);
varDyRetro = varDy  + ( (varVy * (tDt * tDt)) + q);

% filter retrodicted data with historical data */
K = varDyRetro / max(1e-6, (varDyRetro + varDyHist));

dyFilt    = ((1.0 - K) * dyRetro)  +  (K * dyHist);
varDyFilt =  (1.0 - K) * varDyRetro;

== matlab function LM_LIB/LM_OTLBuf1InfoNew/LM_OTL_BufLe1StoreInfoCalc/LM_OTL_ObjSICCurLeObj2InBufLe1/LM_OTL_BufL1DyInfo/MATLAB Function ==
  data: dx input; dyFilt output; dy input; varDy input; vy input; varVy input; psiDt input; tDt input; dyHist input; varDyHist input; varDyFilt output
function  [dyFilt,varDyFilt] = KF_Func(dx,dy,varDy,...
    vy,varVy,psiDt,tDt,dyHist,varDyHist)


ayManeuver = 5;
vyAbs  = vy + (psiDt*dx);


% Calculate process noise: (0.5*a_maneuver*t^2)^2 */
q = (tDt*tDt) * (tDt*tDt);
q =q*(0.5 * ayManeuver)*(0.5 * ayManeuver);
% the following code caused problems on bit-identity: */
% q = (0.5 * CF_TRYFUS_ayManeuver) * (tDt*tDt); */
% q *=q; */

% retrodict current object data */
dyRetro    = dy - (vyAbs  * tDt);
varDyRetro = varDy  + ( (varVy * (tDt * tDt)) + q);

% filter retrodicted data with historical data */
K = varDyRetro / max(1e-6, (varDyRetro + varDyHist));

dyFilt    = ((1.0 - K) * dyRetro)  +  (K * dyHist);
varDyFilt =  (1.0 - K) * varDyRetro;

== matlab function LM_LIB/LM_FusBLPathInfoFilt/LM_Fus_BLFntPathC0Filt/MATLAB Function ==
  data: u1 input; y output; yk1 input
function y = fcn(u1,yk1)
y = single(u1);
if isnan(u1)
    if isnan(yk1)
        y = single(0);
    else
        if yk1 ~= 0
            y = single(yk1);
        else
            y = single(0);
        end
    end
end

== matlab function LM_LIB/LM_FusBLPathInfoFilt/LM_Fus_BLPathC1Filt/MATLAB Function ==
  data: u1 input; y output; yk1 input
function y = fcn(u1,yk1)
y = single(u1);
if isnan(u1)
    if isnan(yk1)
        y = single(0);
    else
        if yk1 ~= 0
            y = single(yk1);
        else
            y = single(0);
        end
    end
end

== matlab function LM_LIB/LM_FusBLPathInfoFilt/LM_Fus_BLPathC2Filt/MATLAB Function ==
  data: u1 input; y output; yk1 input
function y = fcn(u1,yk1)
y = single(u1);
if isnan(u1)
    if isnan(yk1)
        y = single(0);
    else
        if yk1 ~= 0
            y = single(yk1);
        else
            y = single(0);
        end
    end
end

== matlab function LM_LIB/LM_FusBLPathInfoFilt/LM_Fus_BLPath3C3Filt/MATLAB Function ==
  data: u1 input; y output; yk1 input
function y = fcn(u1,yk1)
y = single(u1);
if isnan(u1)
    if isnan(yk1)
        y = single(0);
    else
        if yk1 ~= 0
            y = single(yk1);
        else
            y = single(0);
        end
    end
end

== matlab function LM_LIB/LM_FusBLPathInfoFilt/LM_FusBLPathQuliatyFilt/MATLAB Function ==
  data: u1 input; y output; yk1 input
function y = fcn(u1,yk1)
y = single(u1);
if isnan(u1)
    if isnan(yk1)
        y = single(0);
    else
        if yk1 ~= 0
            y = single(yk1);
        else
            y = single(0);
        end
    end
end
